simulink model "flexible_drive"  (R2021b)
settings: Solver=ode45  StartTime=0.0  StopTime=9  RelTol=1e-3  EnableMultiTasking=on
values from neighbouring files (symbols this model uses):
  b1 = 0.0085    [part4_prelab.m]    (also in simulation_vs_exp.m; simulation_vs_exp_3_1.m; simulation_vs_exp_3_2.m; simulation_vs_exp_3_3.m)
  b2 = 8.4745E-4    (= 0.00084745)    [part4_prelab.m]    (also in simulation_vs_exp.m; simulation_vs_exp_3_1.m; simulation_vs_exp_3_2.m; simulation_vs_exp_3_3.m)
  c = 4.2    [part4_prelab.m]    (also in simulation_vs_exp.m = 0; simulation_vs_exp_3_1.m = 0; simulation_vs_exp_3_2.m = 0; simulation_vs_exp_3_3.m = 0)
  d1 = 0.5934    [simulation_vs_exp_3_1.m]    (also in simulation_vs_exp_3_2.m; simulation_vs_exp_3_3.m)
  d2 = 0.05934    [simulation_vs_exp_3_1.m]    (also in simulation_vs_exp_3_2.m; simulation_vs_exp_3_3.m)
  k = 0.0351    [part4_prelab.m]    (also in simulation_vs_exp.m; simulation_vs_exp_3_1.m; simulation_vs_exp_3_2.m; simulation_vs_exp_3_3.m)
  m1 = 2.6634E-4    (= 0.00026634)    [part4_prelab.m]    (also in simulation_vs_exp.m; simulation_vs_exp_3_1.m; simulation_vs_exp_3_2.m; simulation_vs_exp_3_3.m)
  m2 = 1.4383E-4    (= 0.00014383)    [part4_prelab.m]    (also in simulation_vs_exp.m; simulation_vs_exp_3_1.m; simulation_vs_exp_3_2.m; simulation_vs_exp_3_3.m)
undefined symbols (not defined in the file or in its folder): sgn, Ts
settings Model: Creator=user  LastModifiedBy=parth
settings SolverCC: AlgebraicLoopSolver=TrustRegion
settings DataIOCC: LimitDataPoints=on  SaveFormat=Array  SignalLoggingSaveFormat=ModelDataLogs  ReturnWorkspaceOutputs=off  SignalLoggingName=sigsOut
settings OptimizationCC: LifeSpan=inf
settings DebuggingCC: SaveWithParameterizedLinksMsg=none  UnderspecifiedInitializationDetection=Classic  MergeDetectMultiDrivingBlocksExec=none  SignalResolutionControl=TryResolveAllWithWarning  MultiTaskDSMMsg=warning  MultiTaskCondExecSysMsg=none  SFUnexpectedBacktrackingDiag=warning  SFNoUnconditionalDefaultTransitionDiag=warning  SFMachineParentedDataDiag=warning  ArithmeticOperatorsInVariantConditions=warning
settings HardwareCC: ProdBitPerPointer=32  ProdBitPerSizeT=32  ProdBitPerPtrDiffT=32  ProdLargestAtomicFloat=None  ProdIntDivRoundTo=Undefined  ProdEndianess=Unspecified  ProdWordSize=32  ProdHWDeviceType=32-bit Generic  TargetUnknown=on
settings ModelReferenceCC: PropagateSignalLabelsOutOfModel=off
settings SFSimCC: SimUseLocalCustomCode=off  CustomCodeUndefinedFunction=UseInterfaceOnly
settings RTWCC: RTWUseLocalCustomCode=off
settings CodeAppCC: StateflowObjectComments=on
settings GRTTargetCC: TargetLangStandard=C89/C90 (ANSI)  CombineOutputUpdateFcns=off  GRTInterface=on
settings ConfigComp: CovMetricSettings=dw  CovSaveCumulativeToWorkspaceVar=on  CovSaveSingleToWorkspaceVar=on  CovExternalEMLEnable=off

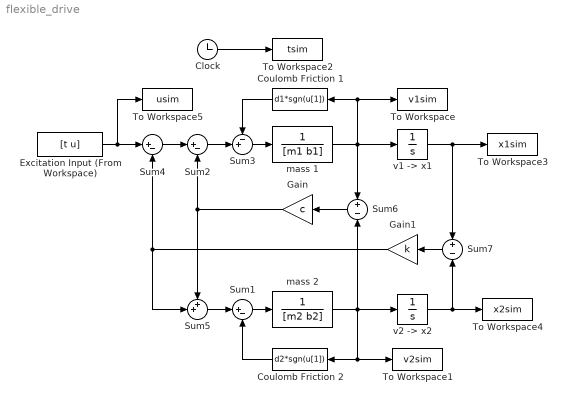
== system flexible_drive ==
  Clock : Clock
  Coulomb Friction 1 : Fcn  Expr=d1*sgn(u[1])
  Coulomb Friction 2 : Fcn  Expr=d2*sgn(u[1])
  Excitation Input (From Workspace) : FromWorkspace  VariableName=[t u]  SampleTime=-1  ZeroCross=off  OutputAfterFinalValue=Holding final value
  Gain : Gain  Gain=c  SaturateOnIntegerOverflow=on  OutDataTypeStr=Inherit: Same as input  ParamDataTypeStr=Inherit: Same as input
  Gain1 : Gain  Gain=k  SaturateOnIntegerOverflow=on  OutDataTypeStr=Inherit: Same as input  ParamDataTypeStr=Inherit: Same as input
  Sum1 : Sum  Inputs=|+-  SaturateOnIntegerOverflow=on
  Sum2 : Sum  Inputs=|+-  SaturateOnIntegerOverflow=on
  Sum3 : Sum  Inputs=-+|  SaturateOnIntegerOverflow=on
  Sum4 : Sum  Inputs=|+-  SaturateOnIntegerOverflow=on
  Sum5 : Sum  Inputs=++|  SaturateOnIntegerOverflow=on
  Sum6 : Sum  Inputs=+|-  SaturateOnIntegerOverflow=on
  Sum7 : Sum  Inputs=+|-  SaturateOnIntegerOverflow=on
  To Workspace : ToWorkspace  VariableName=v1sim  SampleTime=Ts
  To Workspace1 : ToWorkspace  VariableName=v2sim  SampleTime=Ts
  To Workspace2 : ToWorkspace  VariableName=tsim  SampleTime=Ts
  To Workspace3 : ToWorkspace  VariableName=x1sim  SampleTime=Ts
  To Workspace4 : ToWorkspace  VariableName=x2sim  SampleTime=Ts
  To Workspace5 : ToWorkspace  VariableName=usim  SampleTime=Ts
  mass 1 : TransferFcn  Denominator=[m1 b1]
  mass 2 : TransferFcn  Denominator=[m2 b2]
  "v1 -> x1" : Integrator
  "v2 -> x2" : Integrator
  wires:
  mass 1/1 -> "v1 -> x1"/1, Sum6/1, Coulomb Friction 1/1, To Workspace/1
  Clock/1 -> To Workspace2/1
  Sum3/1 -> mass 1/1
  Coulomb Friction 1/1 -> Sum3/1
  mass 2/1 -> "v2 -> x2"/1, Sum6/2, Coulomb Friction 2/1, To Workspace1/1
  Sum1/1 -> mass 2/1
  Coulomb Friction 2/1 -> Sum1/2
  Sum2/1 -> Sum3/2
  Sum5/1 -> Sum1/1
  Sum6/1 -> Gain/1
  Gain/1 -> Sum2/2, Sum5/1
  "v1 -> x1"/1 -> Sum7/1, To Workspace3/1
  "v2 -> x2"/1 -> Sum7/2, To Workspace4/1
  Sum7/1 -> Gain1/1
  Gain1/1 -> Sum4/2, Sum5/2
  Sum4/1 -> Sum2/1
  Excitation Input (From Workspace)/1 -> Sum4/1, To Workspace5/1
